simulink model "Simulink_Model"  (R2024a)
settings: Solver=VariableStepAuto  StartTime=0.0  StopTime=100  RelTol=1e-3
settings Model: Creator=sabyasachi  LastModifiedBy=lenovo
settings ModelReferenceCC: EnableRefExpFcnMdlSchedulingChecks=on
settings RTWCC: GenCodeOnly=on  GPUComputeCapability=3.5

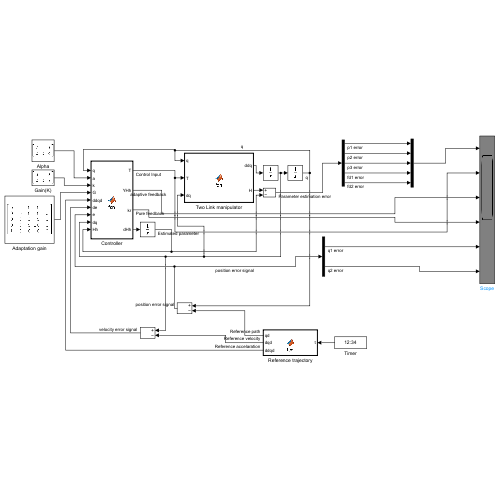
[thumbnail: Simulink's stored preview of the top-level diagram]
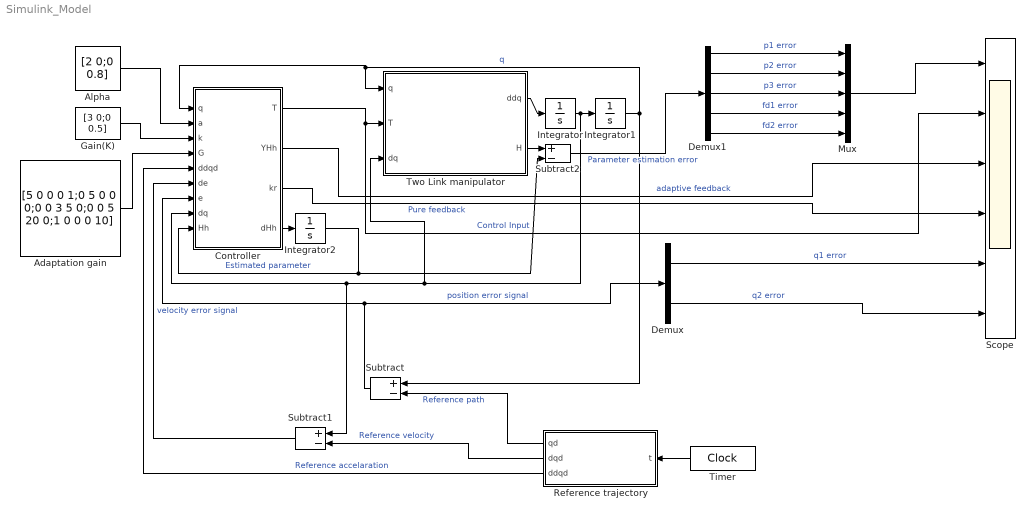
== system Simulink_Model ==
  Adaptation gain : Constant  Value=[5 0 0 0 1;0 5 0 0 0;0 0 3 5 0;0 0 5 20 0;1 0 0 0 10]
  Alpha : Constant  Value=[2 0;0 0.8]
  Controller : MATLAB Function  TreatAsAtomicUnit=on
  Demux : Demux  Outputs=2
  Demux1 : Demux  Outputs=5
  Gain(K) : Constant  Value=[3 0;0 0.5]
  Integrator : Integrator  InitialCondition=[0;0]
  Integrator1 : Integrator  InitialCondition=[0;0]
  Integrator2 : Integrator  InitialCondition=[0;0;0;0;0]
  Mux : Mux  Inputs=5
  Reference trajectory : MATLAB Function  TreatAsAtomicUnit=on
  Scope : Scope  NumInputPorts=6
  Subtract : Sum  Inputs=+-
  Subtract1 : Sum  Inputs=+-
  Subtract2 : Sum  Inputs=+-
  Timer : DigitalClock  SampleTime=0.001
  Two Link manipulator : MATLAB Function  TreatAsAtomicUnit=on
  wires:
  Timer/1 -> Reference trajectory/1(t)
  Integrator1/1 -> Two Link manipulator/1(q), Controller/1(q), Subtract/1  "q"
  Integrator/1 -> Controller/8(dq), Subtract1/1, Two Link manipulator/3(dq), Integrator1/1
  Two Link manipulator/1(ddq) -> Integrator/1
  Reference trajectory/1(qd) -> Subtract/2  "Reference path"
  Reference trajectory/2(dqd) -> Subtract1/2  "Reference velocity"
  Reference trajectory/3(ddqd) -> Controller/5(ddqd)  "Reference accelaration"
  Controller/1(T) -> Scope/2, Two Link manipulator/2(T)  "Control Input"
  Alpha/1 -> Controller/2(a)
  Subtract/1 -> Controller/7(e), Demux/1  "position error signal"
  Subtract1/1 -> Controller/6(de)  "velocity error signal"
  Gain(K)/1 -> Controller/3(k)
  Controller/4(dHh) -> Integrator2/1
  Integrator2/1 -> Subtract2/2, Controller/9(Hh)  "Estimated parameter"
  Adaptation gain/1 -> Controller/4(G)
  Demux/2 -> Scope/6  "q2 error"
  Two Link manipulator/2(H) -> Subtract2/1
  Demux/1 -> Scope/5  "q1 error"
  Subtract2/1 -> Demux1/1  "Parameter estimation error"
  Controller/2(YHh) -> Scope/3  "adaptive feedback"
  Controller/3(kr) -> Scope/4  "Pure feedback"
  Demux1/1 -> Mux/1  "p1 error"
  Demux1/2 -> Mux/2  "p2 error"
  Demux1/3 -> Mux/3  "p3 error"
  Demux1/4 -> Mux/4  "fd1 error"
  Demux1/5 -> Mux/5  "fd2 error"
  Mux/1 -> Scope/1

== matlab function Simulink_Model/Reference trajectory ==
  data: t input; qd output; dqd output; ddqd output
function [qd,dqd,ddqd] = fcn(t)
qd=[(0.5*sin(t));(2*cos(t/4))];
dqd=[0.5*cos(t); -0.5*sin(t/4)];
ddqd=[-0.5*sin(t); -0.125*cos(t/4)]

== matlab function Simulink_Model/Two Link manipulator ==
  data: q input; T input; ddq output; dq input; H output
function [ddq,H] = fcn(q,T,dq)
p=[3.473,0.196,0.242];
F=[5.3 0;0 1.1];
c2=cos(q(2));
s2=sin(q(2));
M=[(p(1)+2*p(3)*c2) (p(2)+p(3)*c2); (p(2)+p(3)*c2) p(2)];
V=[(-p(3)*s2*dq(2)) (-p(3)*s2*(dq(1)+dq(2))); (p(3)*s2*dq(1)) 0];
H=[p';F(1,1);F(2,2)];
ddq=M\(T-V*dq-F*dq);

== matlab function Simulink_Model/Controller ==
  data: q input; a input; k input; G input; ddqd input; de input; e input; dq input; T output; YHh output; kr output; dHh output; Hh input
function [T,YHh,kr,dHh] = fcn(q,a,k,G,ddqd,de,e,dq,Hh)
c2=cos(q(2));
s2=sin(q(2));
r=de+a*e;
y11=a(1,1)*de(1)-ddqd(1);
y12=a(2,2)*de(2)-ddqd(2);
y13=2*c2*a(1,1)*de(1)-2*c2*ddqd(1)+c2*a(2,2)*de(2)-c2*ddqd(2)-s2*dq(2)*r(1)+2*s2*dq(1)*dq(2)-s2*(dq(1)+dq(2))*r(2)+s2*dq(2)*dq(2);
y14=-dq(1);
y22=a(1,1)*de(1)-ddqd(1)+a(2,2)*de(2)-ddqd(2);
y23=c2*a(1,1)*de(1)-c2*ddqd(1)+s2*dq(1)*r(1)-s2*dq(1)*dq(1);
y25=-dq(2);
Y=[y11 y12 y13 y14 0;0 y22 y23 0 y25];
dHh=G*Y'*r;
kr=-k*r;
YHh=-Y*Hh;
T=YHh+kr;
